simulink model "Modele_pendule_e"  (R2020b)
settings: Solver=VariableStepAuto  StartTime=0.0  StopTime=100  RelTol=1e-3
undefined symbols (not defined in the file or in its folder): A_obs, B_obs, C_obs, kd, ki, kp, Kx, L, now, x_0
libraries: pid_lib x1
settings Model: Creator=georgesghazi  LastModifiedBy=georgesghazi

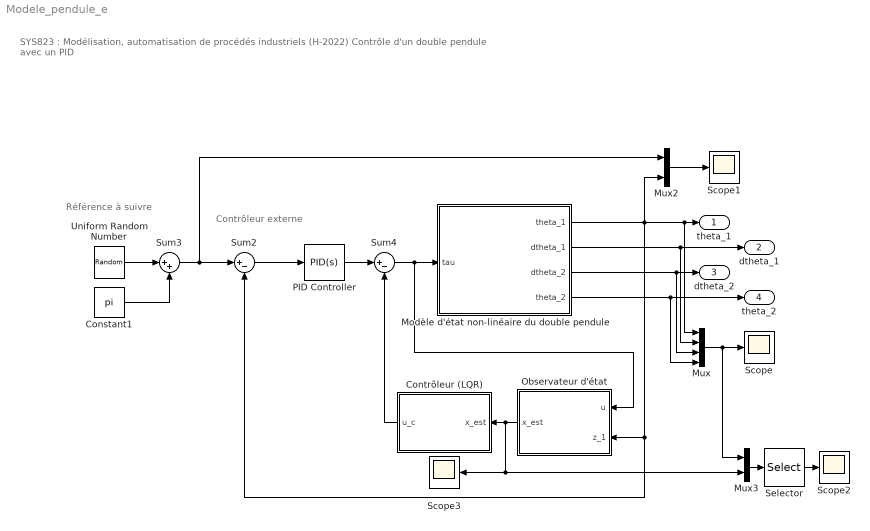
== system Modele_pendule_e ==
  note: Contrôleur externe
  note: Référence à suivre
  note: SYS823 : Modélisation, automatisation de procédés industriels (H-2022)
      |
      | Contrôle d'un double pendule avec un PID
  Constant1 : Constant  Value=pi
  Contrôleur (LQR) : Subsystem
  Modèle d'état non-linéaire du double pendule : Subsystem
  Mux : Mux
  Mux2 : Mux  Inputs=2
  Mux3 : Mux  Inputs=2
  Observateur d'état : Subsystem
  PID Controller : pid_lib/PID Controller  Controller=PID  Form=Parallel  TimeDomain=Continuous-time  UseExternalTs=off  SampleTime=-1  IntegratorMethod=Forward Euler  FilterMethod=Forward Euler  ControllerParametersSource=internal  P=kp  I=ki  D=kd  UseFilter=on  N=100000  TunerSelectOption=Transfer Function Based (PID Tuner App)  InitialConditionSource=internal  InitialConditionForIntegrator=0  InitialConditionForFilter=0  DifferentiatorICPrevScaledInput=0  ExternalReset=none  TrackingMode=off  Kt=1  LimitOutput=off  SatLimitsSource=internal  UpperSaturationLimit=inf  LowerSaturationLimit=-inf  LinearizeAsGain=on  AntiWindupMode=none  Kb=1  POutMin=[]  POutMax=[]  IOutMin=[]  IOutMax=[]  DOutMin=[]  DOutMax=[]  NOutMin=[]  NOutMax=[]  SumOutMin=[]  SumOutMax=[]  SaturationOutMin=[]  SaturationOutMax=[]  PParamMin=[]  PParamMax=[]  IParamMin=[]  IParamMax=[]  DParamMin=[]  DParamMax=[]  NParamMin=[]  NParamMax=[]  KbParamMin=[]  KbParamMax=[]  KtParamMin=[]  KtParamMax=[]  KbOutMin=[]  KbOutMax=[]  KtOutMin=[]  KtOutMax=[]  IntegratorOutMin=[]  IntegratorOutMax=[]  FilterOutMin=[]  FilterOutMax=[]  SumI1OutMin=[]  SumI1OutMax=[]  SumI2OutMin=[]  SumI2OutMax=[]  SumI3OutMin=[]  SumI3OutMax=[]  SumI4OutMin=[]  SumI4OutMax=[]  SumDOutMin=[]  SumDOutMax=[]  DifferentiatorOutMin=[]  DifferentiatorOutMax=[]  FilterDiffOutCoefMin=[]  FilterDiffOutCoefMax=[]  ReciprocalOutMin=[]  ReciprocalOutMax=[]  SumDenOutMin=[]  SumDenOutMax=[]  SumNumOutMin=[]  SumNumOutMax=[]  DivideOutMin=[]  DivideOutMax=[]  UdiffTsProdOutMin=[]  UdiffTsProdOutMax=[]  NTsProdOutMin=[]  NTsProdOutMax=[]  UintegralTsProdOutMin=[]  UintegralTsProdOutMax=[]  UngainTsProdOutMin=[]  UngainTsProdOutMax=[]  IntegratorContinuousStateAttributes=''  IntegratorStateMustResolveToSignalObject=off  IntegratorRTWStateStorageClass=Auto  FilterContinuousStateAttributes=''  FilterStateMustResolveToSignalObject=off  FilterRTWStateStorageClass=Auto  ParallelPVariant=InternalParameters  IdealPVariant=Disabled  IVariant=InternalParameters  DVariant=InternalParameters  IntegratorVariant=Continuous  SatVariant=Disabled  AWVariant=Passthrough  PCopyVariant=Disabled  TRVariant=Disabled  FdbkBlocksVariant=Forward  IdealPFdbkVariant=Disabled  SatFdbkVariant=Disabled  DerivativeFilterVariant=ContFilter  NVariant=InternalParameters  NCopyVariant=Disabled  FilterICVariant=InternalICsFilter  IntegratorICVariant=InternalICs  ExternalResetVariant=Disabled  TRSumVariant=Passthrough  SumFdbkVariant=Disabled  SumVariant=Sum_PID  TsampFilterVariant=InternalTs  TsampNgainVariant=Passthrough  TsampIntegralVariant=Passthrough  ExternalSaturationOutDataTypeStr=Inherit: Same as second input
  Scope{,1..3} (4 alike) : Scope
  Selector : Selector  InputPortWidth=8  IndexOptions=Index vector (dialog)  Indices=[1 5]  OutputSizes=1
  Sum2 : Sum  Inputs=|+-
  Sum3 : Sum  Inputs=|++
  Sum4 : Sum  Inputs=|+-
  Uniform Random Number : UniformRandomNumber  Minimum=-5*pi/180  Maximum=+5*pi/180  Seed=round(now)  SampleTime=20
  theta_1 : Outport
  dtheta_1 : Outport  Port=2
  dtheta_2 : Outport  Port=3
  theta_2 : Outport  Port=4
  wires:
  Mux/1 -> Mux3/1, Scope/1
  Modèle d'état non-linéaire du double pendule/1(theta_1) -> Mux2/2, theta_1/1, Mux/1, Observateur d'état/2(z_1), Sum2/2
  Modèle d'état non-linéaire du double pendule/2(dtheta_1) -> dtheta_1/1, Mux/2
  Modèle d'état non-linéaire du double pendule/3(dtheta_2) -> dtheta_2/1, Mux/3
  Modèle d'état non-linéaire du double pendule/4(theta_2) -> theta_2/1, Mux/4
  Sum4/1 -> Observateur d'état/1(u), Modèle d'état non-linéaire du double pendule/1(tau)
  Sum2/1 -> PID Controller/1
  Sum3/1 -> Sum2/1, Mux2/1
  Uniform Random Number/1 -> Sum3/1
  Constant1/1 -> Sum3/2
  Mux2/1 -> Scope1/1
  PID Controller/1 -> Sum4/1
  Mux3/1 -> Selector/1
  Observateur d'état/1(x_est) -> Scope3/1, Mux3/2, Contrôleur (LQR)/1(x_est)
  Contrôleur (LQR)/1(u_c) -> Sum4/2
  Selector/1 -> Scope2/1

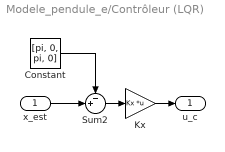
== system Modele_pendule_e/Contrôleur (LQR) ==
  x_est : Inport
  Constant : Constant  Value=[pi, 0, pi, 0]
  Kx : Gain  Gain=Kx  Multiplication=Matrix(K*u) (u vector)
  Sum2 : Sum  Inputs=-+|
  u_c : Outport
  wires:
  Sum2/1 -> Kx/1
  x_est/1 -> Sum2/2
  Constant/1 -> Sum2/1
  Kx/1 -> u_c/1

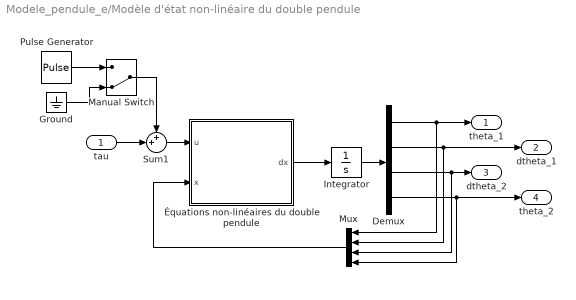
== system Modele_pendule_e/Modèle d'état non-linéaire du double pendule ==
  tau : Inport
  Demux : Demux
  Ground : Ground
  Integrator : Integrator  InitialCondition=x_0
  Manual Switch : ManualSwitch  CurrentSetting=0
  Mux : Mux
  Pulse Generator : DiscretePulseGenerator  PulseType=Time based  Amplitude=5  Period=10  PulseWidth=0.1
  Sum1 : Sum  Inputs=++|
  Équations non-linéaires du double pendule : MATLAB Function  TreatAsAtomicUnit=on
  theta_1 : Outport
  dtheta_1 : Outport  Port=2
  dtheta_2 : Outport  Port=3
  theta_2 : Outport  Port=4
  wires:
  Équations non-linéaires du double pendule/1(dx) -> Integrator/1
  Integrator/1 -> Demux/1
  Demux/2 -> Mux/2, dtheta_1/1
  Demux/4 -> Mux/4, theta_2/1
  Demux/1 -> theta_1/1, Mux/1
  Mux/1 -> Équations non-linéaires du double pendule/2(x)
  Demux/3 -> Mux/3, dtheta_2/1
  Pulse Generator/1 -> Manual Switch/1
  Ground/1 -> Manual Switch/2
  Manual Switch/1 -> Sum1/1
  tau/1 -> Sum1/2
  Sum1/1 -> Équations non-linéaires du double pendule/1(u)

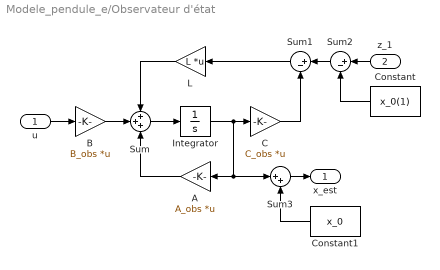
== system Modele_pendule_e/Observateur d'état ==
  u : Inport
  z_1 : Inport  Port=2
  A : Gain  Gain=A_obs  Multiplication=Matrix(K*u) (u vector)
  B : Gain  Gain=B_obs  Multiplication=Matrix(K*u) (u vector)
  C : Gain  Gain=C_obs  Multiplication=Matrix(K*u) (u vector)
  Constant : Constant  Value=x_0(1)
  Constant1 : Constant  Value=x_0
  Integrator : Integrator  InitialCondition=[0, 0, 0.01, 0]
  L : Gain  Gain=L  Multiplication=Matrix(K*u) (u vector)
  Sum : Sum  Inputs=+++
  Sum1 : Sum  Inputs=|+-
  Sum2 : Sum  Inputs=|+-
  Sum3 : Sum  Inputs=|++
  x_est : Outport
  wires:
  u/1 -> B/1
  B/1 -> Sum/2
  Sum/1 -> Integrator/1
  A/1 -> Sum/3
  Integrator/1 -> C/1, Sum3/1, A/1
  L/1 -> Sum/1
  Sum1/1 -> L/1
  C/1 -> Sum1/2
  Sum2/1 -> Sum1/1
  z_1/1 -> Sum2/1
  Sum3/1 -> x_est/1
  Constant1/1 -> Sum3/2
  Constant/1 -> Sum2/2

== matlab function Modele_pendule_e/Modèle d'état non-linéaire du double pendule/Équations non-linéaires du double pendule ==
  data: u input; dx output; x input
function dx = fcn(u, x)
% Déclaration des constantes 
m_1 = 1; m_2 = 1;
l_1 = 2; l_2 = 2;
g_0 = 9.81;

% Calcul de la dérivée du vecteur d'état
dx = zeros(size(x));

dx(1) = x(2);
dx(2) = -(l_1*l_2*m_2*sin(x(1) - x(3))*x(4)^2 - u - l_1*m_2*cos(x(1) - x(3))*(g_0*sin(x(3)) - ...
    l_1*x(2)^2*sin(x(1) - x(3))) + g_0*l_1*m_1*sin(x(1)) + g_0*l_1*m_2*sin(x(1)))/(l_1^2*m_1 + l_1^2*m_2);
dx(3) = x(4);
dx(4) = (l_1*sin(x(1) - x(3))*x(2)^2 - g_0*sin(x(3)) + (l_1*cos(x(1) - x(3))*...
    (l_1*l_2*m_2*sin(x(1) - x(3))*x(4)^2 - u + g_0*l_1*m_1*sin(x(1)) + ...
    g_0*l_1*m_2*sin(x(1))))/(l_1^2*m_1 + l_1^2*m_2))/l_2;
